simulink library "NullStateEstimateBus"  (R2018b)
settings: Solver=VariableStepAuto  StartTime=0.0  StopTime=10.0  RelTol=1e-3
settings Model: Creator=RA24876  LastModifiedBy=RA24876
settings SFSimCC: SimUseLocalCustomCode=off
settings RTWCC: RTWUseLocalCustomCode=off
settings CodeAppCC: StateflowObjectComments=on

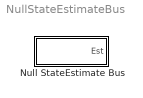
== system NullStateEstimateBus ==
  Null StateEstimate Bus : Subsystem  mask(Null StateEstimate Bus){}
      mask help: Creates a StateEstimate bus signal with all null values. Assign values to elements with a Bus Assignment block.

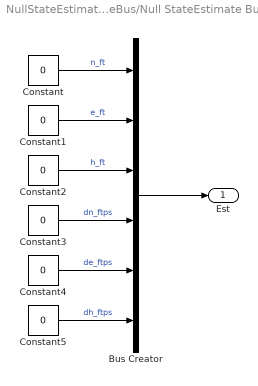
== system NullStateEstimateBus/Null StateEstimate Bus ==
  Bus Creator : BusCreator  Inputs=6  OutDataTypeStr=Bus: StateEstimate
      settings: InheritFromInputs=off
  Constant{,1..5} (6 alike) : Constant  Value=0
  Est : Outport  OutDataTypeStr=Bus: StateEstimate
  wires:
  Constant2/1 -> Bus Creator/3  "h_ft"
  Constant/1 -> Bus Creator/1  "n_ft"
  Constant3/1 -> Bus Creator/4  "dn_ftps"
  Constant5/1 -> Bus Creator/6  "dh_ftps"
  Constant4/1 -> Bus Creator/5  "de_ftps"
  Bus Creator/1 -> Est/1
  Constant1/1 -> Bus Creator/2  "e_ft"
